simulink model "A4b"  (R2018a)
settings: Solver=VariableStepAuto  StartTime=0.0  StopTime=50  RelTol=1e-3
settings Model: Creator=U500304  LastModifiedBy=U500304

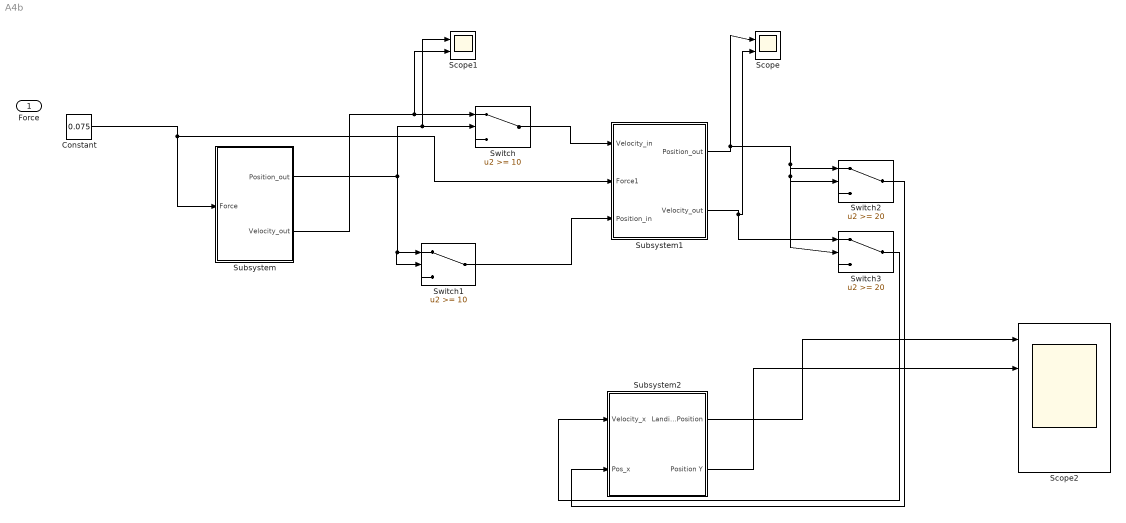
== system A4b ==
  Force : Inport
  Constant : Constant  Value=0.075
  Scope : Scope  NumInputPorts=2
  Scope1 : Scope  NumInputPorts=2
  Scope2 : Scope  NumInputPorts=5
  Subsystem : Subsystem
  Subsystem1 : Subsystem
  Subsystem2 : Subsystem
  Switch : Switch  Threshold=10
  Switch1 : Switch  Threshold=10
  Switch2 : Switch  Threshold=20
  Switch3 : Switch  Threshold=20
  wires:
  Constant/1 -> Subsystem1/2(Force1), Subsystem/1(Force)
  Subsystem1/1(Position_out) -> Switch2/1, Switch3/2, Switch2/2, Scope/1
  Subsystem1/2(Velocity_out) -> Switch3/1, Scope/2
  Subsystem/1(Position_out) -> Switch1/2, Switch1/1, Scope1/1, Switch/2
  Subsystem/2(Velocity_out) -> Scope1/2, Switch/1
  Switch1/1 -> Subsystem1/3(Position_in)
  Switch/1 -> Subsystem1/1("Velocity_in ")
  Switch2/1 -> Subsystem2/2(Pos_x)
  Switch3/1 -> Subsystem2/1(Velocity_x)
  Subsystem2/1(Landing Position) -> Scope2/1
  Subsystem2/2(Position Y) -> Scope2/2

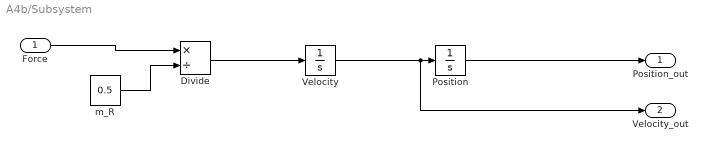
== system A4b/Subsystem ==
  Force : Inport
  Divide : Product  Inputs=*/
  Position : Integrator
  Velocity : Integrator
  m_R : Constant  Value=0.5
  Position_out : Outport
  Velocity_out : Outport  Port=2
  wires:
  Velocity/1 -> Velocity_out/1, Position/1
  Force/1 -> Divide/1
  Divide/1 -> Velocity/1
  m_R/1 -> Divide/2
  Position/1 -> Position_out/1

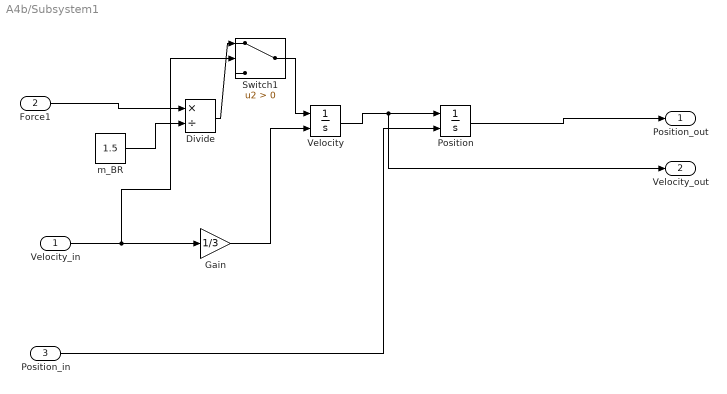
== system A4b/Subsystem1 ==
  "Velocity_in " : Inport
  Force1 : Inport  Port=2
  Position_in : Inport  Port=3
  Divide : Product  Inputs=*/
  Gain : Gain  Gain=1/3
  Position : Integrator  InitialConditionSource=external
  Switch1 : Switch  Criteria=u2 > Threshold
  Velocity : Integrator  InitialConditionSource=external
  m_BR : Constant  Value=1.5
  Position_out : Outport
  Velocity_out : Outport  Port=2
  wires:
  Position_in/1 -> Position/2
  Force1/1 -> Divide/1
  m_BR/1 -> Divide/2
  Position/1 -> Position_out/1
  Divide/1 -> Switch1/1
  Gain/1 -> Velocity/2
  "Velocity_in "/1 -> Switch1/2, Gain/1
  Switch1/1 -> Velocity/1
  Velocity/1 -> Velocity_out/1, Position/1

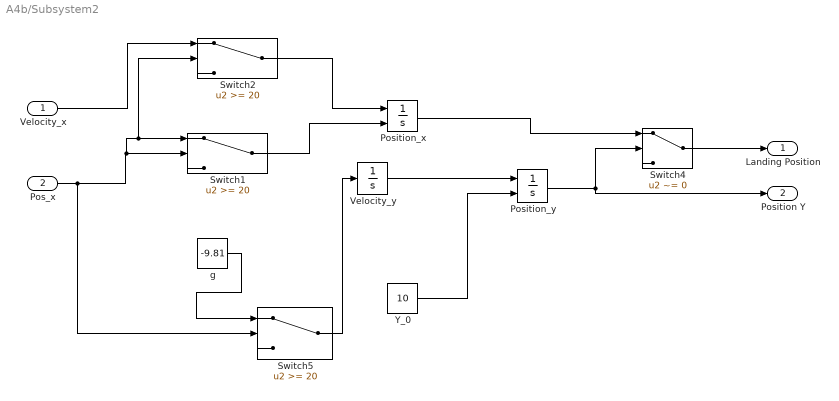
== system A4b/Subsystem2 ==
  Velocity_x : Inport
  Pos_x : Inport  Port=2
  Position_x : Integrator  InitialConditionSource=external
  Position_y : Integrator  InitialConditionSource=external  InitialCondition=10
  Switch1 : Switch  Threshold=20
  Switch2 : Switch  Threshold=20
  Switch4 : Switch  Criteria=u2 ~= 0
  Switch5 : Switch  Threshold=20
  Velocity_y : Integrator
  Y_0 : Constant  Value=10
  g : Constant  Value=-9.81
  Landing Position : Outport
  Position Y : Outport  Port=2
  wires:
  Switch5/1 -> Velocity_y/1
  Position_x/1 -> Switch4/1
  Pos_x/1 -> Switch2/2, Switch1/1, Switch1/2, Switch5/2
  Switch4/1 -> Landing Position/1
  g/1 -> Switch5/1
  Velocity_y/1 -> Position_y/1
  Y_0/1 -> Position_y/2
  Position_y/1 -> Position Y/1, Switch4/2
  Switch1/1 -> Position_x/2
  Velocity_x/1 -> Switch2/1
  Switch2/1 -> Position_x/1
